simulink model "proba"  (R2014b)
settings: Solver=ode45  StartTime=0.0  StopTime=20.0  RelTol=1e-3
libraries: simulink x1
settings Model: Creator=nina  LastModifiedBy=nina

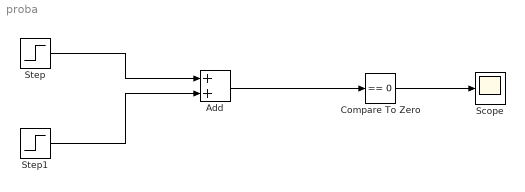
== system proba ==
  Add : Sum
  Compare To Zero : simulink/Logic and Bit Operations/Compare To Zero  relop===  OutDataTypeStr=boolean
  Scope : Scope
  Step : Step  SampleTime=0.01
  Step1 : Step  Time=10  After=-1  SampleTime=0.01
  wires:
  Compare To Zero/1 -> Scope/1
  Add/1 -> Compare To Zero/1
  Step/1 -> Add/1
  Step1/1 -> Add/2
